simulink model "DrvStFtIsPosChk"  (R2018b)
settings: Solver=FixedStepDiscrete  StartTime=0.0  StopTime=10.0  FixedStep=0.01  RelTol=1e-3
undefined symbols (not defined in the file or in its folder): KeSMSuFirstRwStFootrestPosDelta_Val, KeSMSuFirstRwStFootrestPosTolr_Val
libraries: StIsPosChkLib x6, simulink x5
settings Model: ModifiedHistory="2023.9.14 V2.1.0  Bug 540886 相同问题： 修改VIP模式判断到位的条件为10ms周期计算"  Creator=sn2xws  LastModifiedBy=sn2xws
settings DataIOCC: SaveFormat=StructureWithTime
settings OptimizationCC: DefaultParameterBehavior=Inlined  EnhancedBackFolding=on  PassReuseOutputArgsAs=Individual arguments  ZeroExternalMemoryAtStartup=off  ZeroInternalMemoryAtStartup=off  OptimizeBlockOrder=speed  DifferentSizesBufferReuse=on  OptimizationCustomize=off
settings DebuggingCC: ParameterTunabilityLossMsg=error
settings ModelReferenceCC: ModelReferenceNumInstancesAllowed=Single
settings SFSimCC: MATLABDynamicMemAlloc=off
settings RTWCC: SystemTargetFile=autosar.tlc  GenCodeOnly=on  TemplateMakefile=ert_default_tmf  Description=AUTOSAR  GenerateReport=on  IncludeHyperlinkInReport=on  LaunchReport=on  GenerateTraceInfo=on  GenerateTraceReport=on  GenerateTraceReportSl=on  GenerateTraceReportSf=on  GenerateTraceReportEml=on  GenerateCodeMetricsReport=on
settings CodeAppCC: ForceParamTrailComments=on  IgnoreCustomStorageClasses=off  OperatorAnnotations=on  SimulinkDataObjDesc=on  SFDataObjDesc=on  InsertBlockDesc=on
settings STFCustomTargetCC: TargetLangStandard=C99 (ISO)  MultiwordLength=256  ParMdlRefBuildCompliant=on  CompOptLevelCompliant=on  IncludeMdlTerminateFcn=off  CombineOutputUpdateFcns=on  SuppressErrorStatus=on  ERTCustomFileBanners=on  SupportNonFinite=off  SupportComplex=off  SupportContinuousTime=off  SupportNonInlinedSFcns=off  RemoveResetFunc=on  MATLABClassNameForMDSCustomization=Simulink.SoftwareTarget.ERTCustomization  AutosarCompliant=on  UseToolchainInfoCompliant=on  LookupTableObjectStructAxisOrder=2,1,3,4,...  LUTObjectStructOrderEvenSpacing=Size,Table,Breakpoints  SystemTargetFile=autosar.tlc
settings ERTTargetCC: TargetLangStandard=C99 (ISO)  ConcurrentExecutionCompliant=off  IncludeMdlTerminateFcn=off  SuppressErrorStatus=on  SupportNonFinite=off  SupportComplex=off  ModelStepFunctionPrototypeControlCompliant=off  CPPClassGenCompliant=off  AutosarCompliant=on  LookupTableObjectStructAxisOrder=2,1,3,4,...  LUTObjectStructOrderEvenSpacing=Size,Table,Breakpoints  InlinedParameterPlacement=NonHierarchical  ERTCustomFileTemplate=example_file_process.tlc  ERTFilePackagingFormat=Compact

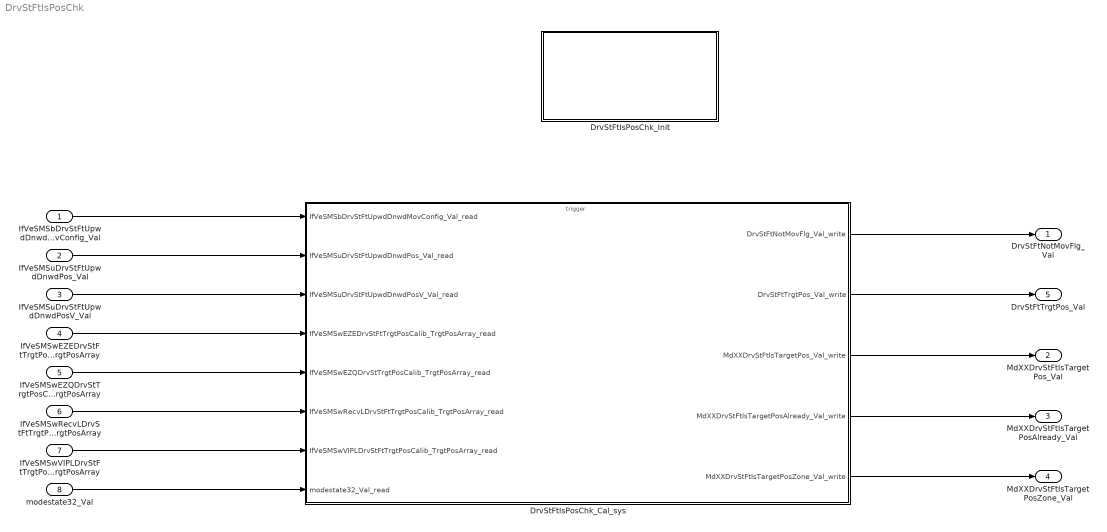
== system DrvStFtIsPosChk ==
  IfVeSMSbDrvStFtUpwdDnwdMovConfig_Val : Inport  OutDataTypeStr=boolean  PortDimensions=1
  IfVeSMSuDrvStFtUpwdDnwdPos_Val : Inport  Port=2  OutDataTypeStr=uint16  PortDimensions=1
  IfVeSMSuDrvStFtUpwdDnwdPosV_Val : Inport  Port=3  OutDataTypeStr=boolean  PortDimensions=1
  IfVeSMSwEZEDrvStFtTrgtPosCalib_TrgtPosArray : Inport  Description=|  Port=4  OutDataTypeStr=uint16  PortDimensions=3
      | 0:Pos
      | 1:Max
      | 2:Min
  IfVeSMSwEZQDrvStTrgtPosCalib_TrgtPosArray : Inport  Description=|  Port=5  OutDataTypeStr=uint16  PortDimensions=3
      | 0:Pos
      | 1:Max
      | 2:Min
  IfVeSMSwRecvLDrvStFtTrgtPosCalib_TrgtPosArray : Inport  Description=|  Port=6  OutDataTypeStr=uint16  PortDimensions=3
      | 0:Pos
      | 1:Max
      | 2:Min
  IfVeSMSwVIPLDrvStFtTrgtPosCalib_TrgtPosArray : Inport  Description=|  Port=7  OutDataTypeStr=uint16  PortDimensions=3
      | 0:Pos
      | 1:Max
      | 2:Min
  modestate32_Val : Inport  Port=8  OutDataTypeStr=uint32  PortDimensions=1
  DrvStFtIsPosChk_Cal_sys : Subsystem
  DrvStFtIsPosChk_Init : Subsystem
  DrvStFtNotMovFlg_Val : Outport  OutDataTypeStr=boolean  PortDimensions=1
  MdXXDrvStFtIsTargetPos_Val : Outport  Port=2  OutDataTypeStr=uint32  PortDimensions=1
  MdXXDrvStFtIsTargetPosAlready_Val : Outport  Port=3  OutDataTypeStr=uint32  PortDimensions=1
  MdXXDrvStFtIsTargetPosZone_Val : Outport  Port=4  OutDataTypeStr=uint32  PortDimensions=1
  DrvStFtTrgtPos_Val : Outport  Port=5  OutDataTypeStr=uint16  PortDimensions=1
  wires:
  DrvStFtIsPosChk_Cal_sys/1(DrvStFtNotMovFlg_Val_write) -> DrvStFtNotMovFlg_Val/1
  DrvStFtIsPosChk_Cal_sys/3(MdXXDrvStFtIsTargetPos_Val_write) -> MdXXDrvStFtIsTargetPos_Val/1
  DrvStFtIsPosChk_Cal_sys/2(DrvStFtTrgtPos_Val_write) -> DrvStFtTrgtPos_Val/1
  DrvStFtIsPosChk_Cal_sys/4(MdXXDrvStFtIsTargetPosAlready_Val_write) -> MdXXDrvStFtIsTargetPosAlready_Val/1
  DrvStFtIsPosChk_Cal_sys/5(MdXXDrvStFtIsTargetPosZone_Val_write) -> MdXXDrvStFtIsTargetPosZone_Val/1
  IfVeSMSbDrvStFtUpwdDnwdMovConfig_Val/1 -> DrvStFtIsPosChk_Cal_sys/1(IfVeSMSbDrvStFtUpwdDnwdMovConfig_Val_read)
  IfVeSMSuDrvStFtUpwdDnwdPos_Val/1 -> DrvStFtIsPosChk_Cal_sys/2(IfVeSMSuDrvStFtUpwdDnwdPos_Val_read)
  IfVeSMSuDrvStFtUpwdDnwdPosV_Val/1 -> DrvStFtIsPosChk_Cal_sys/3(IfVeSMSuDrvStFtUpwdDnwdPosV_Val_read)
  IfVeSMSwEZEDrvStFtTrgtPosCalib_TrgtPosArray/1 -> DrvStFtIsPosChk_Cal_sys/4(IfVeSMSwEZEDrvStFtTrgtPosCalib_TrgtPosArray_read)
  IfVeSMSwEZQDrvStTrgtPosCalib_TrgtPosArray/1 -> DrvStFtIsPosChk_Cal_sys/5(IfVeSMSwEZQDrvStTrgtPosCalib_TrgtPosArray_read)
  IfVeSMSwRecvLDrvStFtTrgtPosCalib_TrgtPosArray/1 -> DrvStFtIsPosChk_Cal_sys/6(IfVeSMSwRecvLDrvStFtTrgtPosCalib_TrgtPosArray_read)
  IfVeSMSwVIPLDrvStFtTrgtPosCalib_TrgtPosArray/1 -> DrvStFtIsPosChk_Cal_sys/7(IfVeSMSwVIPLDrvStFtTrgtPosCalib_TrgtPosArray_read)
  modestate32_Val/1 -> DrvStFtIsPosChk_Cal_sys/8(modestate32_Val_read)

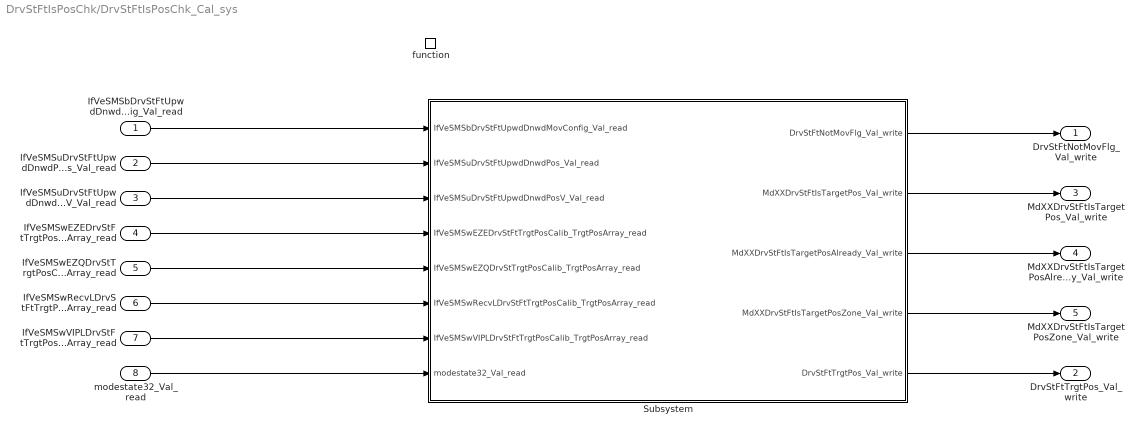
== system DrvStFtIsPosChk/DrvStFtIsPosChk_Cal_sys ==
  IfVeSMSbDrvStFtUpwdDnwdMovConfig_Val_read : Inport
  IfVeSMSuDrvStFtUpwdDnwdPos_Val_read : Inport  Port=2
  IfVeSMSuDrvStFtUpwdDnwdPosV_Val_read : Inport  Port=3
  IfVeSMSwEZEDrvStFtTrgtPosCalib_TrgtPosArray_read : Inport  Port=4
  IfVeSMSwEZQDrvStTrgtPosCalib_TrgtPosArray_read : Inport  Port=5
  IfVeSMSwRecvLDrvStFtTrgtPosCalib_TrgtPosArray_read : Inport  Port=6
  IfVeSMSwVIPLDrvStFtTrgtPosCalib_TrgtPosArray_read : Inport  Port=7
  modestate32_Val_read : Inport  Port=8
  function : TriggerPort  TriggerType=function-call  IsSimulinkFunction=on  FunctionName=DrvStFtIsPosChk_Cal  VariantControl=(inherit)
  Subsystem : Subsystem
  DrvStFtNotMovFlg_Val_write : Outport
      settings: EnsureOutportIsVirtual=on
  DrvStFtTrgtPos_Val_write : Outport  Port=2
      settings: EnsureOutportIsVirtual=on
  MdXXDrvStFtIsTargetPos_Val_write : Outport  Port=3
      settings: EnsureOutportIsVirtual=on
  MdXXDrvStFtIsTargetPosAlready_Val_write : Outport  Port=4
      settings: EnsureOutportIsVirtual=on
  MdXXDrvStFtIsTargetPosZone_Val_write : Outport  Port=5
      settings: EnsureOutportIsVirtual=on
  wires:
  Subsystem/1(DrvStFtNotMovFlg_Val_write) -> DrvStFtNotMovFlg_Val_write/1
  Subsystem/5(DrvStFtTrgtPos_Val_write) -> DrvStFtTrgtPos_Val_write/1
  Subsystem/4(MdXXDrvStFtIsTargetPosZone_Val_write) -> MdXXDrvStFtIsTargetPosZone_Val_write/1
  Subsystem/3(MdXXDrvStFtIsTargetPosAlready_Val_write) -> MdXXDrvStFtIsTargetPosAlready_Val_write/1
  Subsystem/2(MdXXDrvStFtIsTargetPos_Val_write) -> MdXXDrvStFtIsTargetPos_Val_write/1
  IfVeSMSbDrvStFtUpwdDnwdMovConfig_Val_read/1 -> Subsystem/1(IfVeSMSbDrvStFtUpwdDnwdMovConfig_Val_read)
  IfVeSMSuDrvStFtUpwdDnwdPos_Val_read/1 -> Subsystem/2(IfVeSMSuDrvStFtUpwdDnwdPos_Val_read)
  IfVeSMSuDrvStFtUpwdDnwdPosV_Val_read/1 -> Subsystem/3(IfVeSMSuDrvStFtUpwdDnwdPosV_Val_read)
  IfVeSMSwEZEDrvStFtTrgtPosCalib_TrgtPosArray_read/1 -> Subsystem/4(IfVeSMSwEZEDrvStFtTrgtPosCalib_TrgtPosArray_read)
  IfVeSMSwEZQDrvStTrgtPosCalib_TrgtPosArray_read/1 -> Subsystem/5(IfVeSMSwEZQDrvStTrgtPosCalib_TrgtPosArray_read)
  IfVeSMSwRecvLDrvStFtTrgtPosCalib_TrgtPosArray_read/1 -> Subsystem/6(IfVeSMSwRecvLDrvStFtTrgtPosCalib_TrgtPosArray_read)
  IfVeSMSwVIPLDrvStFtTrgtPosCalib_TrgtPosArray_read/1 -> Subsystem/7(IfVeSMSwVIPLDrvStFtTrgtPosCalib_TrgtPosArray_read)
  modestate32_Val_read/1 -> Subsystem/8(modestate32_Val_read)

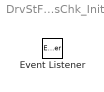
== system DrvStFtIsPosChk/DrvStFtIsPosChk_Init ==
  Event Listener : EventListener  EventName=reset

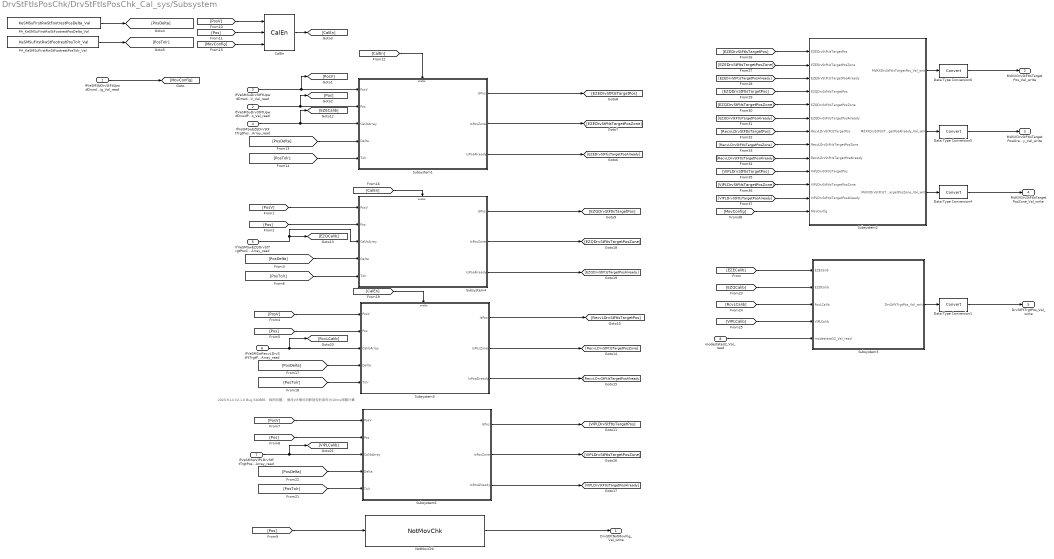
== system DrvStFtIsPosChk/DrvStFtIsPosChk_Cal_sys/Subsystem ==
  note: 2023.9.14 V2.1.0 Bug 540886 相同问题： 修改VIP模式判断到位的条件为10ms周期计算
  IfVeSMSbDrvStFtUpwdDnwdMovConfig_Val_read : Inport
  IfVeSMSuDrvStFtUpwdDnwdPos_Val_read : Inport  Port=2
  IfVeSMSuDrvStFtUpwdDnwdPosV_Val_read : Inport  Port=3
  IfVeSMSwEZEDrvStFtTrgtPosCalib_TrgtPosArray_read : Inport  Port=4
  IfVeSMSwEZQDrvStTrgtPosCalib_TrgtPosArray_read : Inport  Port=5
  IfVeSMSwRecvLDrvStFtTrgtPosCalib_TrgtPosArray_read : Inport  Port=6
  IfVeSMSwVIPLDrvStFtTrgtPosCalib_TrgtPosArray_read : Inport  Port=7
  modestate32_Val_read : Inport  Port=8
  CalEn : StIsPosChkLib/CalEn  SystemSampleTime=-1
  Data Type Conversion{1,4..6} (4 alike) : DataTypeConversion
  NotMovChk : StIsPosChkLib/NotMovChk  SystemSampleTime=-1
  PA_KeSMSuFirstRwStFootrestPosDelta_Val : Constant  Value=KeSMSuFirstRwStFootrestPosDelta_Val
  PA_KeSMSuFirstRwStFootrestPosTolr_Val : Constant  Value=KeSMSuFirstRwStFootrestPosTolr_Val
  Subsystem1 : Subsystem
  Subsystem2 : Subsystem
  Subsystem3 : Subsystem
  Subsystem4 : Subsystem
  Subsystem5 : Subsystem
  Subsystem6 : Subsystem
  DrvStFtNotMovFlg_Val_write : Outport
      settings: EnsureOutportIsVirtual=on
  MdXXDrvStFtIsTargetPos_Val_write : Outport  Port=2
      settings: EnsureOutportIsVirtual=on
  MdXXDrvStFtIsTargetPosAlready_Val_write : Outport  Port=3
      settings: EnsureOutportIsVirtual=on
  MdXXDrvStFtIsTargetPosZone_Val_write : Outport  Port=4
      settings: EnsureOutportIsVirtual=on
  DrvStFtTrgtPos_Val_write : Outport  Port=5
      settings: EnsureOutportIsVirtual=on
  wires:
  [CalEn] -> Subsystem1/Enable
  [PosV] -> CalEn/1
  [EZQDrvStFtIsTargetPos] -> Subsystem2/4(EZQDrvStFtIsTargetPos)
  Subsystem1/1(IsPos) -> [EZEDrvStFtIsTargetPos]
  Subsystem4/1(IsPos) -> [EZQDrvStFtIsTargetPos]
  Data Type Conversion6/1 -> MdXXDrvStFtIsTargetPos_Val_write/1
  IfVeSMSwRecvLDrvStFtTrgtPosCalib_TrgtPosArray_read/1 -> Subsystem5/3(CalibArray), [RcvLCalib]
  [RcvLCalib] -> Subsystem3/3(RcvLCalib)
  IfVeSMSuDrvStFtUpwdDnwdPos_Val_read/1 -> [Pos], Subsystem1/2(Pos)
  [VIPLDrvStFtIsTargetPosAlready] -> Subsystem2/12(VIPLDrvStFtIsTargetPosAlready)
  [Pos] -> Subsystem4/2(Pos)
  [EZEDrvStFtisTargetPosAlready] -> Subsystem2/3(EZEDrvStFtIsTargetPosAlready)
  [Pos] -> Subsystem6/2(Pos)
  IfVeSMSwEZEDrvStFtTrgtPosCalib_TrgtPosArray_read/1 -> Subsystem1/3(CalibArray), [EZECalib]
  [EZEDrvStFtIsTargetPosZone] -> Subsystem2/2(EZEDrvStFtIsTargetPosZone)
  [PosV] -> Subsystem4/1(PosV)
  CalEn/1 -> [CalEn]
  Subsystem5/1(IsPos) -> [RecvLDrvStFtIsTargetPos]
  IfVeSMSwEZQDrvStTrgtPosCalib_TrgtPosArray_read/1 -> Subsystem4/3(CalibArray), [EZQCalib]
  [PosTolr] -> Subsystem1/5(Tolr)
  [EZEDrvStFtIsTargetPos] -> Subsystem2/1(EZEDrvStFtIsTargetPos)
  NotMovChk/1 -> DrvStFtNotMovFlg_Val_write/1
  Subsystem5/2(IsPosZone) -> [RecvLDrvStFtIsTargetPosZone]
  PA_KeSMSuFirstRwStFootrestPosTolr_Val/1 -> [PosTolr]
  [MovConfig] -> CalEn/3
  Subsystem1/2(IsPosZone) -> [EZEDrvStFtIsTargetPosZone]
  IfVeSMSbDrvStFtUpwdDnwdMovConfig_Val_read/1 -> [MovConfig]
  [Pos] -> NotMovChk/1
  PA_KeSMSuFirstRwStFootrestPosDelta_Val/1 -> [PosDelta]
  [PosDelta] -> Subsystem1/4(Delta)
  [PosTolr] -> Subsystem6/5(Tolr)
  [PosDelta] -> Subsystem5/4(Delta)
  [PosV] -> Subsystem6/1(PosV)
  [EZQDrvStFtIsTargetPosAlready] -> Subsystem2/6(EZQDrvStFtIsTargetPosAlready)
  [Pos] -> Subsystem5/2(Pos)
  IfVeSMSwVIPLDrvStFtTrgtPosCalib_TrgtPosArray_read/1 -> Subsystem6/3(CalibArray), [VIPLCalib]
  [PosTolr] -> Subsystem5/5(Tolr)
  Subsystem6/2(IsPosZone) -> [VIPLDrvStFtIsTargetPosZone]
  Data Type Conversion5/1 -> MdXXDrvStFtIsTargetPosAlready_Val_write/1
  Subsystem2/1(MdXXDrvStFtIsTargetPos_Val_write) -> Data Type Conversion6/1
  [PosTolr] -> Subsystem4/5(Tolr)
  [VIPLCalib] -> Subsystem3/4(VIPLCalib)
  [PosDelta] -> Subsystem4/4(Delta)
  [CalEn] -> Subsystem4/Enable
  [VIPLDrvStFtIsTargetPos] -> Subsystem2/10(VIPLDrvStFtIsTargetPos)
  [RecvLDrvStFtIsTargetPos] -> Subsystem2/7(RecvLDrvStFtIsTargetPos)
  [PosV] -> Subsystem5/1(PosV)
  Subsystem4/2(IsPosZone) -> [EZQDrvStFtIsTargetPosZone]
  [EZQDrvStFtIsTargetPosZone] -> Subsystem2/5(EZQDrvStFtIsTargetPosZone)
  Subsystem6/1(IsPos) -> [VIPLDrvStFtIsTargetPos]
  [EZECalib] -> Subsystem3/1(EZECalib)
  [EZQCalib] -> Subsystem3/2(EZQCalib)
  Subsystem2/2(MdXXDrvStFtIsTargetPosAlready_Val_write) -> Data Type Conversion5/1
  Subsystem5/3(IsPosAlready) -> [RecvLDrvStFtIsTargetPosAlready]
  Subsystem6/3(IsPosAlready) -> [VIPLDrvStFtIsTargetPosAlready]
  Subsystem2/3(MdXXDrvStFtIsTargetPosZone_Val_write) -> Data Type Conversion4/1
  [RecvLDrvStFtIsTargetPosZone] -> Subsystem2/8(RecvLDrvStFtIsTargetPosZone)
  [VIPLDrvStFtIsTargetPosZone] -> Subsystem2/11(VIPLDrvStFtIsTargetPosZone)
  [CalEn] -> Subsystem5/Enable
  [PosDelta] -> Subsystem6/4(Delta)
  [Pos] -> CalEn/2
  [MovConfig] -> Subsystem2/13(MovConfig)
  [RecvLDrvStFtIsTargetPosAlready] -> Subsystem2/9(RecvLDrvStFtIsTargetPosAlready)
  IfVeSMSuDrvStFtUpwdDnwdPosV_Val_read/1 -> Subsystem1/1(PosV), [PosV]
  Subsystem1/3(IsPosAlready) -> [EZEDrvStFtisTargetPosAlready]
  modestate32_Val_read/1 -> Subsystem3/5(modestate32_Val_read)
  Data Type Conversion1/1 -> DrvStFtTrgtPos_Val_write/1
  Subsystem4/3(IsPosAlready) -> [EZQDrvStFtIsTargetPosAlready]
  Data Type Conversion4/1 -> MdXXDrvStFtIsTargetPosZone_Val_write/1
  Subsystem3/1(DrvStFtTrgtPos_Val_write) -> Data Type Conversion1/1

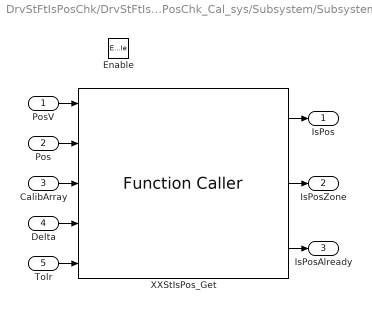
== system DrvStFtIsPosChk/DrvStFtIsPosChk_Cal_sys/Subsystem/Subsystem1 ==
  PosV : Inport
  Pos : Inport  Port=2
  CalibArray : Inport  Port=3
  Delta : Inport  Port=4
  Tolr : Inport  Port=5
  Enable : EnablePort
  XXStIsPos_Get : FunctionCaller  FunctionPrototype=[IsPos,IsPosZone,IsPosAlready] = XXStIsPos_Get(PosV,Pos,CalibArray,Delta,Tolr)  InputArgumentSpecifications=boolean(true), uint16(1), uint16([1;1;1]), uint16(1), uint16(1)  OutputArgumentSpecifications=boolean(true), boolean(true), boolean(true)
  IsPos : Outport
  IsPosZone : Outport  Port=2
  IsPosAlready : Outport  Port=3
  wires:
  PosV/1 -> XXStIsPos_Get/1
  Delta/1 -> XXStIsPos_Get/4
  CalibArray/1 -> XXStIsPos_Get/3
  XXStIsPos_Get/1 -> IsPos/1
  XXStIsPos_Get/2 -> IsPosZone/1
  Pos/1 -> XXStIsPos_Get/2
  XXStIsPos_Get/3 -> IsPosAlready/1
  Tolr/1 -> XXStIsPos_Get/5

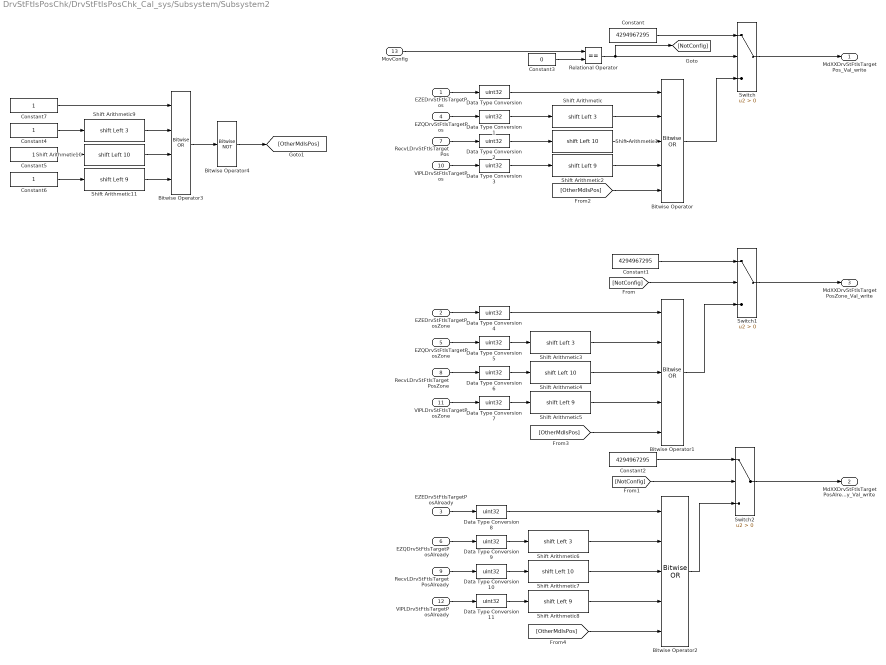
== system DrvStFtIsPosChk/DrvStFtIsPosChk_Cal_sys/Subsystem/Subsystem2 ==
  EZEDrvStFtIsTargetPos : Inport
  EZEDrvStFtIsTargetPosZone : Inport  Port=2
  EZEDrvStFtIsTargetPosAlready : Inport  Port=3
  EZQDrvStFtIsTargetPos : Inport  Port=4
  EZQDrvStFtIsTargetPosZone : Inport  Port=5
  EZQDrvStFtIsTargetPosAlready : Inport  Port=6
  RecvLDrvStFtIsTargetPos : Inport  Port=7
  RecvLDrvStFtIsTargetPosZone : Inport  Port=8
  RecvLDrvStFtIsTargetPosAlready : Inport  Port=9
  VIPLDrvStFtIsTargetPos : Inport  Port=10
  VIPLDrvStFtIsTargetPosZone : Inport  Port=11
  VIPLDrvStFtIsTargetPosAlready : Inport  Port=12
  MovConfig : Inport  Port=13
  Bitwise Operator : simulink/Logic and Bit Operations/Bitwise Operator  logicop=OR  UseBitMask=off  NumInputPorts=5  BitMask=bin2dec('11011001')  BitMaskRealWorld=Stored Integer
  Bitwise Operator1 : simulink/Logic and Bit Operations/Bitwise Operator  logicop=OR  UseBitMask=off  NumInputPorts=5  BitMask=bin2dec('11011001')  BitMaskRealWorld=Stored Integer
  Bitwise Operator2 : simulink/Logic and Bit Operations/Bitwise Operator  logicop=OR  UseBitMask=off  NumInputPorts=5  BitMask=bin2dec('11011001')  BitMaskRealWorld=Stored Integer
  Bitwise Operator3 : simulink/Logic and Bit Operations/Bitwise Operator  logicop=OR  UseBitMask=off  NumInputPorts=4  BitMask=bin2dec('11011001')  BitMaskRealWorld=Stored Integer
  Bitwise Operator4 : simulink/Logic and Bit Operations/Bitwise Operator  logicop=NOT  UseBitMask=off  BitMask=bin2dec('11011001')  BitMaskRealWorld=Stored Integer
  Constant : Constant  Value=4294967295  OutDataTypeStr=uint32
  Constant1 : Constant  Value=4294967295  OutDataTypeStr=uint32
  Constant2 : Constant  Value=4294967295  OutDataTypeStr=uint32
  Constant3 : Constant  Value=0  OutDataTypeStr=uint8
  Constant{4..7} (4 alike) : Constant  OutDataTypeStr=uint32
  Data Type Conversion{,1..11} (12 alike) : DataTypeConversion  OutDataTypeStr=uint32
  Relational Operator : RelationalOperator  Operator===  OutDataTypeStr=boolean  RndMeth=Simplest
  Shift Arithmetic{,3,6,9} (4 alike) : ArithShift  BitShiftNumber=3  BitShiftDirection=Left
  Shift Arithmetic{1,4,7,10} (4 alike) : ArithShift  BitShiftNumber=10  BitShiftDirection=Left
  Shift Arithmetic{2,5,8,11} (4 alike) : ArithShift  BitShiftNumber=9  BitShiftDirection=Left
  Switch : Switch  Criteria=u2 > Threshold
  Switch1 : Switch  Criteria=u2 > Threshold
  Switch2 : Switch  Criteria=u2 > Threshold
  MdXXDrvStFtIsTargetPos_Val_write : Outport
      settings: EnsureOutportIsVirtual=on
  MdXXDrvStFtIsTargetPosAlready_Val_write : Outport  Port=2
      settings: EnsureOutportIsVirtual=on
  MdXXDrvStFtIsTargetPosZone_Val_write : Outport  Port=3
      settings: EnsureOutportIsVirtual=on
  wires:
  Switch/1 -> MdXXDrvStFtIsTargetPos_Val_write/1
  Relational Operator/1 -> [NotConfig], Switch/2
  Constant/1 -> Switch/1
  [NotConfig] -> Switch1/2
  MovConfig/1 -> Relational Operator/1
  Constant1/1 -> Switch1/1
  Constant2/1 -> Switch2/1
  [NotConfig] -> Switch2/2
  EZEDrvStFtIsTargetPos/1 -> Data Type Conversion/1
  EZQDrvStFtIsTargetPos/1 -> Data Type Conversion1/1
  VIPLDrvStFtIsTargetPos/1 -> Data Type Conversion3/1
  RecvLDrvStFtIsTargetPos/1 -> Data Type Conversion2/1
  Shift Arithmetic1/1 -> Bitwise Operator/3
  Shift Arithmetic2/1 -> Bitwise Operator/4
  Bitwise Operator1/1 -> Switch1/3
  Bitwise Operator2/1 -> Switch2/3
  Data Type Conversion1/1 -> Shift Arithmetic/1
  Data Type Conversion2/1 -> Shift Arithmetic1/1
  Data Type Conversion3/1 -> Shift Arithmetic2/1
  Data Type Conversion7/1 -> Shift Arithmetic5/1
  Data Type Conversion6/1 -> Shift Arithmetic4/1
  Data Type Conversion5/1 -> Shift Arithmetic3/1
  Data Type Conversion4/1 -> Bitwise Operator1/1
  Shift Arithmetic5/1 -> Bitwise Operator1/4
  Shift Arithmetic4/1 -> Bitwise Operator1/3
  Shift Arithmetic3/1 -> Bitwise Operator1/2
  RecvLDrvStFtIsTargetPosZone/1 -> Data Type Conversion6/1
  VIPLDrvStFtIsTargetPosZone/1 -> Data Type Conversion7/1
  EZQDrvStFtIsTargetPosZone/1 -> Data Type Conversion5/1
  EZEDrvStFtIsTargetPosZone/1 -> Data Type Conversion4/1
  Shift Arithmetic6/1 -> Bitwise Operator2/2
  Shift Arithmetic7/1 -> Bitwise Operator2/3
  Shift Arithmetic8/1 -> Bitwise Operator2/4
  Data Type Conversion8/1 -> Bitwise Operator2/1
  Data Type Conversion9/1 -> Shift Arithmetic6/1
  Data Type Conversion10/1 -> Shift Arithmetic7/1
  Data Type Conversion11/1 -> Shift Arithmetic8/1
  EZEDrvStFtIsTargetPosAlready/1 -> Data Type Conversion8/1
  EZQDrvStFtIsTargetPosAlready/1 -> Data Type Conversion9/1
  RecvLDrvStFtIsTargetPosAlready/1 -> Data Type Conversion10/1
  VIPLDrvStFtIsTargetPosAlready/1 -> Data Type Conversion11/1
  Data Type Conversion/1 -> Bitwise Operator/1
  Shift Arithmetic/1 -> Bitwise Operator/2
  Bitwise Operator/1 -> Switch/3
  Switch2/1 -> MdXXDrvStFtIsTargetPosAlready_Val_write/1
  Switch1/1 -> MdXXDrvStFtIsTargetPosZone_Val_write/1
  Constant3/1 -> Relational Operator/2
  Constant4/1 -> Shift Arithmetic9/1
  Constant6/1 -> Shift Arithmetic11/1
  Constant5/1 -> Shift Arithmetic10/1
  Shift Arithmetic9/1 -> Bitwise Operator3/2
  Shift Arithmetic10/1 -> Bitwise Operator3/3
  Shift Arithmetic11/1 -> Bitwise Operator3/4
  Constant7/1 -> Bitwise Operator3/1
  Bitwise Operator3/1 -> Bitwise Operator4/1
  Bitwise Operator4/1 -> [OtherMdIsPos]
  [OtherMdIsPos] -> Bitwise Operator/5
  [OtherMdIsPos] -> Bitwise Operator1/5
  [OtherMdIsPos] -> Bitwise Operator2/5

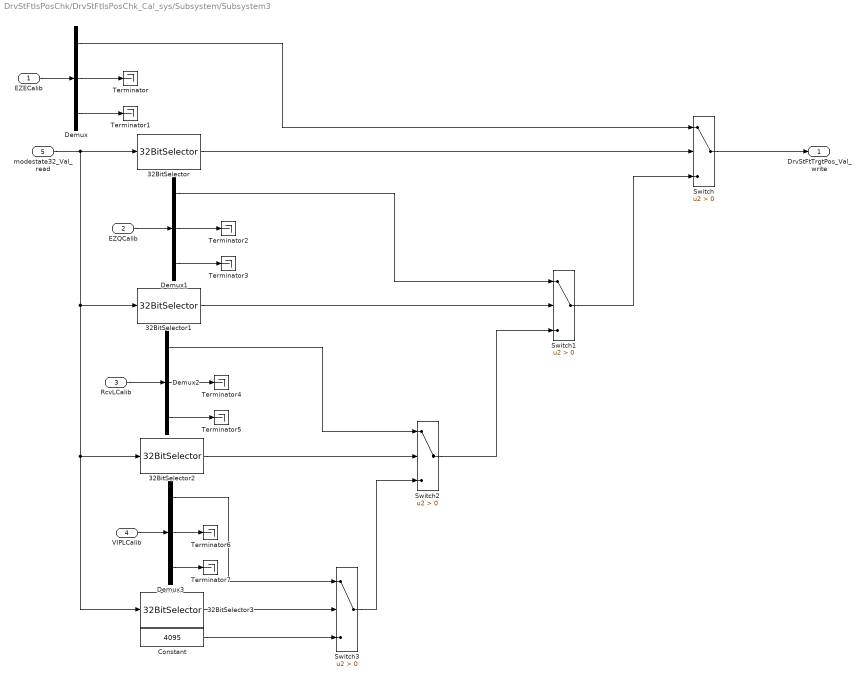
== system DrvStFtIsPosChk/DrvStFtIsPosChk_Cal_sys/Subsystem/Subsystem3 ==
  EZECalib : Inport
  EZQCalib : Inport  Port=2
  RcvLCalib : Inport  Port=3
  VIPLCalib : Inport  Port=4
  modestate32_Val_read : Inport  Port=5
  32BitSelector : StIsPosChkLib/32BitSelector  BitNum=0
  32BitSelector1 : StIsPosChkLib/32BitSelector  BitNum=3
  32BitSelector2 : StIsPosChkLib/32BitSelector  BitNum=10
  32BitSelector3 : StIsPosChkLib/32BitSelector  BitNum=9
  Constant : Constant  Value=4095  OutDataTypeStr=uint16
  Demux{,1..3} (4 alike) : Demux  Outputs=3
  Switch{,1..3} (4 alike) : Switch  Criteria=u2 > Threshold
  Terminator{,1..7} (8 alike) : Terminator
  DrvStFtTrgtPos_Val_write : Outport
      settings: EnsureOutportIsVirtual=on
  wires:
  EZECalib/1 -> Demux/1
  Demux/3 -> Terminator1/1
  Demux/2 -> Terminator/1
  Demux1/2 -> Terminator2/1
  Demux1/3 -> Terminator3/1
  EZQCalib/1 -> Demux1/1
  Demux2/3 -> Terminator5/1
  Demux2/2 -> Terminator4/1
  RcvLCalib/1 -> Demux2/1
  VIPLCalib/1 -> Demux3/1
  Demux3/2 -> Terminator6/1
  Demux3/3 -> Terminator7/1
  modestate32_Val_read/1 -> 32BitSelector3/1, 32BitSelector2/1, 32BitSelector1/1, 32BitSelector/1
  32BitSelector/1 -> Switch/2
  Demux/1 -> Switch/1
  Switch/1 -> DrvStFtTrgtPos_Val_write/1
  Switch1/1 -> Switch/3
  32BitSelector1/1 -> Switch1/2
  Demux1/1 -> Switch1/1
  Switch2/1 -> Switch1/3
  32BitSelector2/1 -> Switch2/2
  Demux2/1 -> Switch2/1
  Switch3/1 -> Switch2/3
  32BitSelector3/1 -> Switch3/2
  Demux3/1 -> Switch3/1
  Constant/1 -> Switch3/3

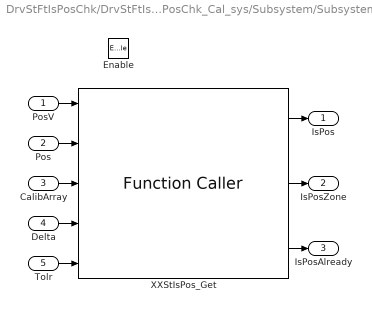
== system DrvStFtIsPosChk/DrvStFtIsPosChk_Cal_sys/Subsystem/Subsystem4 ==
  PosV : Inport
  Pos : Inport  Port=2
  CalibArray : Inport  Port=3
  Delta : Inport  Port=4
  Tolr : Inport  Port=5
  Enable : EnablePort
  XXStIsPos_Get : FunctionCaller  FunctionPrototype=[IsPos,IsPosZone,IsPosAlready] = XXStIsPos_Get(PosV,Pos,CalibArray,Delta,Tolr)  InputArgumentSpecifications=boolean(true), uint16(1), uint16([1;1;1]), uint16(1), uint16(1)  OutputArgumentSpecifications=boolean(true), boolean(true), boolean(true)
  IsPos : Outport
  IsPosZone : Outport  Port=2
  IsPosAlready : Outport  Port=3
  wires:
  Tolr/1 -> XXStIsPos_Get/5
  XXStIsPos_Get/3 -> IsPosAlready/1
  Pos/1 -> XXStIsPos_Get/2
  XXStIsPos_Get/2 -> IsPosZone/1
  XXStIsPos_Get/1 -> IsPos/1
  CalibArray/1 -> XXStIsPos_Get/3
  Delta/1 -> XXStIsPos_Get/4
  PosV/1 -> XXStIsPos_Get/1

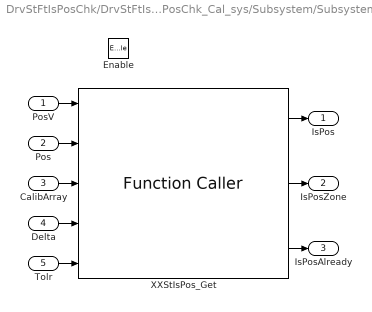
== system DrvStFtIsPosChk/DrvStFtIsPosChk_Cal_sys/Subsystem/Subsystem5 ==
  PosV : Inport
  Pos : Inport  Port=2
  CalibArray : Inport  Port=3
  Delta : Inport  Port=4
  Tolr : Inport  Port=5
  Enable : EnablePort
  XXStIsPos_Get : FunctionCaller  FunctionPrototype=[IsPos,IsPosZone,IsPosAlready] = XXStIsPos_Get(PosV,Pos,CalibArray,Delta,Tolr)  InputArgumentSpecifications=boolean(true), uint16(1), uint16([1;1;1]), uint16(1), uint16(1)  OutputArgumentSpecifications=boolean(true), boolean(true), boolean(true)
  IsPos : Outport
  IsPosZone : Outport  Port=2
  IsPosAlready : Outport  Port=3
  wires:
  PosV/1 -> XXStIsPos_Get/1
  Delta/1 -> XXStIsPos_Get/4
  CalibArray/1 -> XXStIsPos_Get/3
  XXStIsPos_Get/1 -> IsPos/1
  XXStIsPos_Get/2 -> IsPosZone/1
  Pos/1 -> XXStIsPos_Get/2
  XXStIsPos_Get/3 -> IsPosAlready/1
  Tolr/1 -> XXStIsPos_Get/5

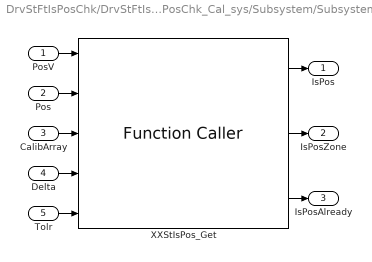
== system DrvStFtIsPosChk/DrvStFtIsPosChk_Cal_sys/Subsystem/Subsystem6 ==
  PosV : Inport
  Pos : Inport  Port=2
  CalibArray : Inport  Port=3
  Delta : Inport  Port=4
  Tolr : Inport  Port=5
  XXStIsPos_Get : FunctionCaller  FunctionPrototype=[IsPos,IsPosZone,IsPosAlready] = XXStIsPos_Get(PosV,Pos,CalibArray,Delta,Tolr)  InputArgumentSpecifications=boolean(true), uint16(1), uint16([1;1;1]), uint16(1), uint16(1)  OutputArgumentSpecifications=boolean(true), boolean(true), boolean(true)
  IsPos : Outport
  IsPosZone : Outport  Port=2
  IsPosAlready : Outport  Port=3
  wires:
  Tolr/1 -> XXStIsPos_Get/5
  XXStIsPos_Get/3 -> IsPosAlready/1
  Pos/1 -> XXStIsPos_Get/2
  XXStIsPos_Get/2 -> IsPosZone/1
  XXStIsPos_Get/1 -> IsPos/1
  CalibArray/1 -> XXStIsPos_Get/3
  Delta/1 -> XXStIsPos_Get/4
  PosV/1 -> XXStIsPos_Get/1
